simulink model "GHV_open_VarialbeMass_elliposid_toolbox"  (R2023b)
settings: Solver=FixedStepAuto  StartTime=0.0  StopTime=10  FixedStep=0.01  MaxStep=0.001  RelTol=1e-3
InitFcn:
  | run('init.m')
values from neighbouring files (symbols this model uses):
  GHV_cfg = struct()    [GHV_Configuration.m]
undefined symbols (not defined in the file or in its folder): Earth, WGS84
libraries: simulink_extras x3, aerolibasang x3, aerolibtransform2 x2, aerolib6dof2 x1, aerolibatmos2 x1, matrix_library x1, aerolibgravity2 x1
settings Model: SimulationMode=accelerator  Creator=Admin  LastModifiedBy=Admin
settings SolverCC: AllowMultiTaskInputOutput=on  ZeroCrossControl=EnableAll  ZeroCrossAlgorithm=Adaptive  AutoInsertRateTranBlk=on
settings DebuggingCC: IgnoredZcDiagnostic=none

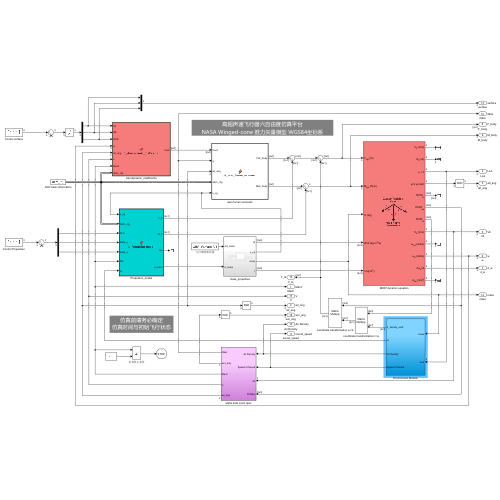
[thumbnail: Simulink's stored preview of the top-level diagram]
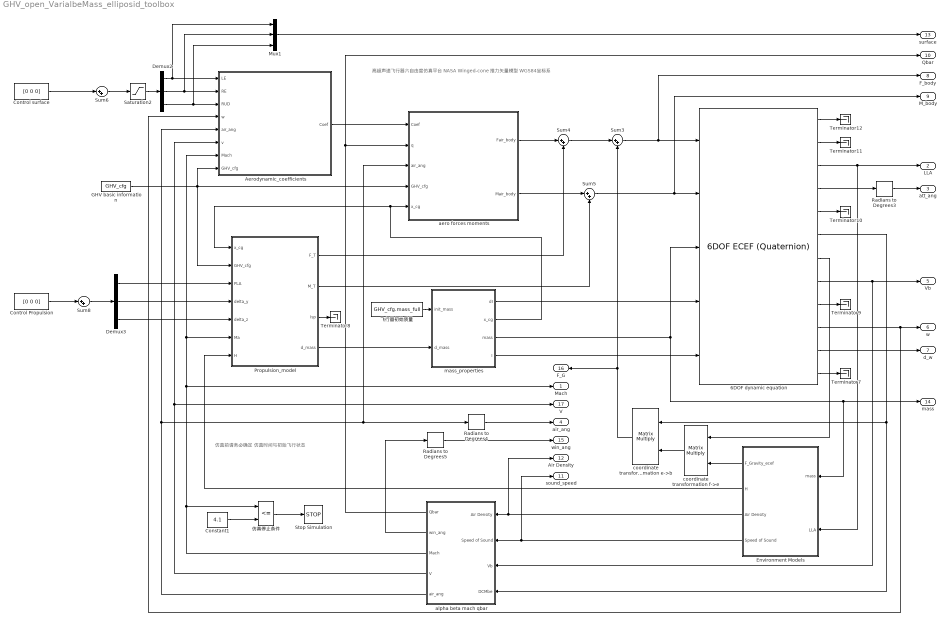
== system GHV_open_VarialbeMass_elliposid_toolbox ==
  note: 高超声速飞行器六自由度仿真平台
      | NASA Winged-cone 推力矢量模型 WGS84坐标系
  note: 仿真前请务必确定
      | 仿真时间与初始飞行状态
  6DOF dynamic equation : aerolib6dof2/6DOF ECEF (Quaternion)  units=Metric (MKS)  mtype=Custom Variable  xg_0=LLA_init  Vm_0=Speed_init  eul_0=Euler_init  pm_0=Omega_init  mass_0=1.0  mass_e=0.5  mass_f=2.0  inertia=eye(3)  inertia_e=eye(3)  inertia_f=2*eye(3)  vre_flag=off  abi_flag=off  ptype=Earth (WGS84)  R=6378137  F=1/298.257223563  w_E=7292115e-11  angle_in=Internal  LPM0=0  quat_statename=''  pm_statename=''  Vm_statename=''  posfixedframe_statename=''  posinertial_statename=''  LPM_statename=''  mass_statename=''
      settings: LibrarySourceBlock=|
      | aerolib6dof2/Custom Variable Mass 6DOF
      | ECEF (Quaternion)
  Aerodynamic_coefficients : MATLAB Function  TreatAsAtomicUnit=on
  Constant1 : Constant  Value=4.1
  Control Propulsion : Constant  Value=[0 0 0]
  Control surface : Constant  Value=[0 0 0]
  Demux2 : Demux  Outputs=3
  Demux3 : Demux  Outputs=3
  Environment Models : Subsystem
  GHV basic information : Constant  Value=GHV_cfg  VectorParams1D=off  OutDataTypeStr=Bus: slBus1
  Mux1 : Mux  Inputs=3
  Propulsion_model : MATLAB Function  TreatAsAtomicUnit=on
  Radians to Degrees3 : simulink_extras/Transformations/Radians to Degrees
  Radians to Degrees4 : simulink_extras/Transformations/Radians to Degrees
  Radians to Degrees5 : simulink_extras/Transformations/Radians to Degrees
  Saturation2 : Saturate  UpperLimit=20  LowerLimit=-20  ZeroCross=off
  Stop Simulation : Stop
  Sum{3..6,8} (5 alike) : Sum  Inputs=|++
  Terminator{7..12} (6 alike) : Terminator
  aero forces moments : MATLAB Function  TreatAsAtomicUnit=on
  alpha beta mach qbar : Subsystem
  coordinate transformation e->b : Product  Multiplication=Matrix(*)
  coordinate transformation f->e : Product  Multiplication=Matrix(*)
  mass_properties : Subsystem
  仿真停止条件 : RelationalOperator  Operator=<=  OutDataTypeStr=boolean  RndMeth=Simplest  InputSameDT=off
  飞行器初始质量 : Constant  Value=GHV_cfg.mass_full
  Mach : Outport  SignalName=Mach
  LLA : Outport  Port=2  SignalName=LLA
  att_ang : Outport  Port=3  SignalName=att_ang
  air_ang : Outport  Port=4  SignalName=air_ang
  Vb : Outport  Port=5  SignalName=Vb
  w : Outport  Port=6  SignalName=w
  d_w : Outport  Port=7  SignalName=d_w
  F_body : Outport  Port=8  SignalName=F_body
  M_body : Outport  Port=9  SignalName=M_body
  Qbar : Outport  Port=10  SignalName=Qbar
  sound_speed : Outport  Port=11  SignalName=sound_speed
  Air Density : Outport  Port=12  SignalName=Air Density
  surface : Outport  Port=13  SignalName=surface
  mass : Outport  Port=14  SignalName=mass
  win_ang : Outport  Port=15  SignalName=win_ang
  F_G : Outport  Port=16  SignalName=F_G
  V : Outport  Port=17  SignalName=V
  wires:
  mass_properties/4(I) -> 6DOF dynamic equation/5
  Propulsion_model/3(Isp) -> Terminator8/1
  alpha beta mach qbar/2(win_ang) -> Radians to Degrees5/1
  Propulsion_model/4(d_mass) -> mass_properties/2(d_mass)
  飞行器初始质量/1 -> mass_properties/1(init_mass)
  仿真停止条件/1 -> Stop Simulation/1
  Demux2/3 -> Aerodynamic_coefficients/3(RUD), Mux1/3
  6DOF dynamic equation/5 -> Terminator10/1
  coordinate transformation e->b/1 -> Sum3/2, F_G/1
  GHV basic information/1 -> aero forces moments/4(GHV_cfg), Propulsion_model/2(GHV_cfg), Aerodynamic_coefficients/8(GHV_cfg)
  6DOF dynamic equation/3 -> LLA/1, Environment Models/2(LLA)
  6DOF dynamic equation/2 -> Terminator11/1
  Environment Models/3(Air Density) -> Air Density/1, alpha beta mach qbar/1(Air Density)
  6DOF dynamic equation/4 -> Radians to Degrees3/1
  Sum8/1 -> Demux3/1
  Demux3/1 -> Propulsion_model/3(PLA)
  alpha beta mach qbar/3(Mach) -> Aerodynamic_coefficients/7(Mach), Propulsion_model/6(Ma), Mach/1, 仿真停止条件/1
  6DOF dynamic equation/8 -> Vb/1, alpha beta mach qbar/3(Vb)
  6DOF dynamic equation/11 -> d_w/1
  Sum4/1 -> Sum3/1
  6DOF dynamic equation/6 -> alpha beta mach qbar/4(DCMbe), coordinate transformation e->b/1
  Propulsion_model/2(M_T) -> Sum5/2
  Sum5/1 -> 6DOF dynamic equation/2, M_body/1
  6DOF dynamic equation/10 -> w/1, Aerodynamic_coefficients/4(w)
  Environment Models/1(F_Gravity_ecef) -> coordinate transformation f->e/2
  mass_properties/1(dI) -> 6DOF dynamic equation/4
  Demux2/1 -> Aerodynamic_coefficients/1(LE), Mux1/1
  Radians to Degrees5/1 -> win_ang/1
  Saturation2/1 -> Demux2/1
  Aerodynamic_coefficients/1(Coef) -> aero forces moments/1(Coef)
  mass_properties/3(mass) -> 6DOF dynamic equation/3, Environment Models/1(mass), mass/1
  Constant1/1 -> 仿真停止条件/2
  Control surface/1 -> Sum6/1
  Sum3/1 -> 6DOF dynamic equation/1, F_body/1
  Radians to Degrees4/1 -> air_ang/1
  alpha beta mach qbar/4(V) -> Aerodynamic_coefficients/6(v), V/1
  alpha beta mach qbar/1(Qbar) -> aero forces moments/2(q), Qbar/1
  Environment Models/2(H) -> Propulsion_model/7(H)
  Demux3/2 -> Propulsion_model/4(delta_y)
  Demux2/2 -> Aerodynamic_coefficients/2(RE), Mux1/2
  6DOF dynamic equation/12 -> Terminator7/1
  Control Propulsion/1 -> Sum8/1
  coordinate transformation f->e/1 -> coordinate transformation e->b/2
  Demux3/3 -> Propulsion_model/5(delta_z)
  Sum6/1 -> Saturation2/1
  Mux1/1 -> surface/1
  Propulsion_model/1(F_T) -> Sum4/2
  aero forces moments/1(Fair_body) -> Sum4/1
  6DOF dynamic equation/9 -> Terminator9/1
  6DOF dynamic equation/7 -> coordinate transformation f->e/1
  aero forces moments/2(Mair_body) -> Sum5/1
  Radians to Degrees3/1 -> att_ang/1
  mass_properties/2(x_cg) -> aero forces moments/5(x_cg), Propulsion_model/1(x_cg)
  Environment Models/4(Speed of Sound) -> sound_speed/1, alpha beta mach qbar/2(Speed of Sound)
  6DOF dynamic equation/1 -> Terminator12/1
  alpha beta mach qbar/5(air_ang) -> Aerodynamic_coefficients/5(air_ang), aero forces moments/3(air_ang), Radians to Degrees4/1

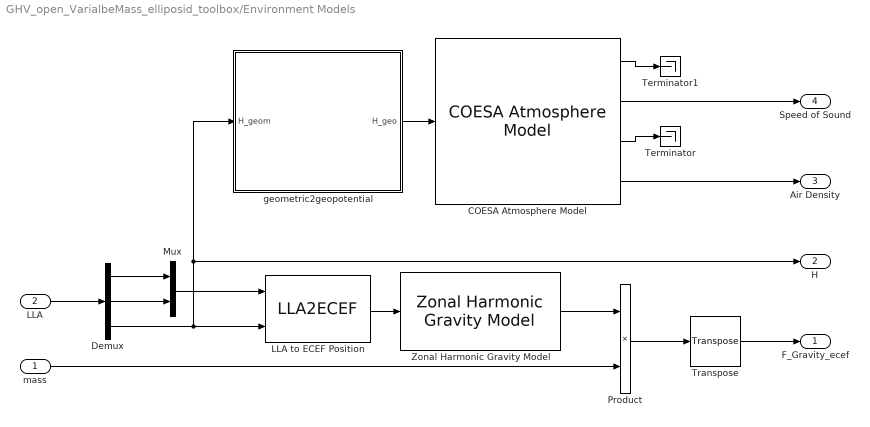
== system GHV_open_VarialbeMass_elliposid_toolbox/Environment Models ==
  mass : Inport
  LLA : Inport  Port=2
  COESA Atmosphere Model : aerolibatmos2/COESA Atmosphere Model  units=Metric (MKS)  spec=1976 COESA-extended U.S. Standard Atmosphere  model=Profile  profile_var=High temperature  profile_percent=1%  profile_alt=5 km (16404 ft)  envelope_var=High temperature  envelope_percent=1%  action=Warning
  Demux : Demux  Outputs=3
  LLA to ECEF Position : LLA2ECEF
  Mux : Mux  Inputs=2
  Product : Product
  Terminator : Terminator
  Terminator1 : Terminator
  Transpose : matrix_library/Transpose
  Zonal Harmonic Gravity Model : aerolibgravity2/Zonal Harmonic Gravity Model  units=Metric (MKS)  degree=2  action=Warning  ptype=Earth  R=6378136.3  GM=398600441500000  jvalue=[1.0826269e-03 -2.5323000e-06 -1.6204000e-06]
  geometric2geopotential : MATLAB Function  TreatAsAtomicUnit=on
  F_Gravity_ecef : Outport
  H : Outport  Port=2
  Air Density : Outport  Port=3
  Speed of Sound : Outport  Port=4
  wires:
  COESA Atmosphere Model/1 -> Terminator1/1
  COESA Atmosphere Model/2 -> Speed of Sound/1
  COESA Atmosphere Model/3 -> Terminator/1
  COESA Atmosphere Model/4 -> Air Density/1
  LLA to ECEF Position/1 -> Zonal Harmonic Gravity Model/1
  Mux/1 -> LLA to ECEF Position/1
  Demux/3 -> geometric2geopotential/1(H_geom), H/1, LLA to ECEF Position/2
  Demux/1 -> Mux/1
  Demux/2 -> Mux/2
  LLA/1 -> Demux/1
  mass/1 -> Product/2
  Zonal Harmonic Gravity Model/1 -> Product/1
  Product/1 -> Transpose/1
  Transpose/1 -> F_Gravity_ecef/1
  geometric2geopotential/1(H_geo) -> COESA Atmosphere Model/1

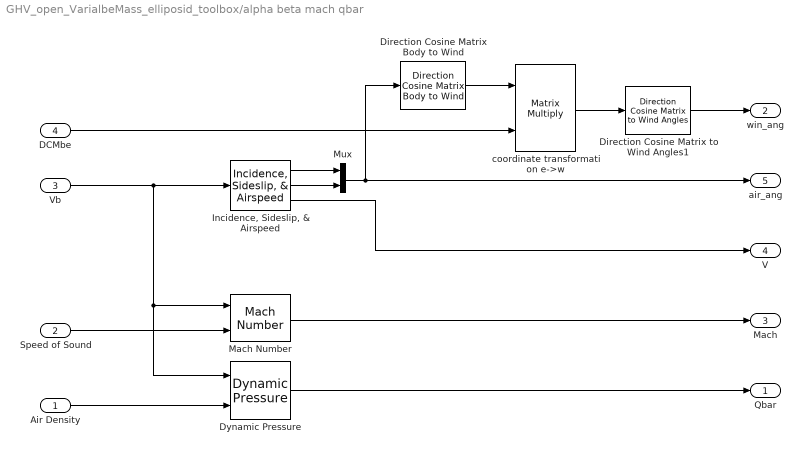
== system GHV_open_VarialbeMass_elliposid_toolbox/alpha beta mach qbar ==
  Air Density : Inport
  Speed of Sound : Inport  Port=2
  Vb : Inport  Port=3
  DCMbe : Inport  Port=4
  Direction Cosine Matrix Body to Wind : aerolibtransform2/Direction Cosine Matrix Body to Wind
  Direction Cosine Matrix to Wind Angles1 : aerolibtransform2/Direction Cosine Matrix to Wind Angles  action=None  tolerance=eps(2)
  Dynamic Pressure : aerolibasang/Dynamic Pressure
  "Incidence, Sideslip, & Airspeed" : aerolibasang/Incidence, Sideslip, & Airspeed
  Mach Number : aerolibasang/Mach Number
  Mux : Mux  Inputs=2
  coordinate transformation e->w : Product  Multiplication=Matrix(*)
  Qbar : Outport
  win_ang : Outport  Port=2
  Mach : Outport  Port=3
  V : Outport  Port=4
  air_ang : Outport  Port=5
  wires:
  Speed of Sound/1 -> Mach Number/2
  Mach Number/1 -> Mach/1
  "Incidence, Sideslip, & Airspeed"/2 -> Mux/2
  Vb/1 -> Dynamic Pressure/1, Mach Number/1, "Incidence, Sideslip, & Airspeed"/1
  Dynamic Pressure/1 -> Qbar/1
  Mux/1 -> Direction Cosine Matrix Body to Wind/1, air_ang/1
  "Incidence, Sideslip, & Airspeed"/1 -> Mux/1
  Air Density/1 -> Dynamic Pressure/2
  "Incidence, Sideslip, & Airspeed"/3 -> V/1
  DCMbe/1 -> coordinate transformation e->w/2
  Direction Cosine Matrix Body to Wind/1 -> coordinate transformation e->w/1
  coordinate transformation e->w/1 -> Direction Cosine Matrix to Wind Angles1/1
  Direction Cosine Matrix to Wind Angles1/1 -> win_ang/1

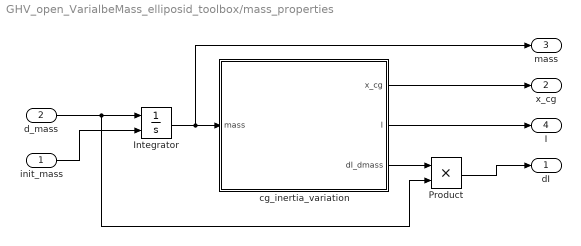
== system GHV_open_VarialbeMass_elliposid_toolbox/mass_properties ==
  init_mass : Inport
  d_mass : Inport  Port=2
  Integrator : Integrator  InitialConditionSource=external
  Product : Product
  cg_inertia_variation : MATLAB Function  TreatAsAtomicUnit=on
  dI : Outport
  x_cg : Outport  Port=2
  mass : Outport  Port=3
  I : Outport  Port=4
  wires:
  Integrator/1 -> mass/1, cg_inertia_variation/1(mass)
  init_mass/1 -> Integrator/2
  cg_inertia_variation/3(dI_dmass) -> Product/1
  d_mass/1 -> Product/2, Integrator/1
  cg_inertia_variation/2(I) -> I/1
  cg_inertia_variation/1(x_cg) -> x_cg/1
  Product/1 -> dI/1

== matlab function GHV_open_VarialbeMass_elliposid_toolbox/Aerodynamic_coefficients ==
  data: LE input; Coef output; RE input; RUD input; w input; air_ang input; v input; Mach input; GHV_cfg input
function Coef = S_Aerodynamic_coefficients(LE, RE, RUD, w, air_ang,v, Mach, GHV_cfg)
    Coef = zeros(6, 1);
    Coef = Aerodynamic_coefficients(LE, RE, RUD, air_ang, v, w, Mach, GHV_cfg);
    Coef = [1;1;1;1;1;1].*Coef;

end

== matlab function GHV_open_VarialbeMass_elliposid_toolbox/Environment Models/geometric2geopotential ==
  data: H_geom input; H_geo output
function H_geo = S_geometric2geopotential(H_geom)

    H_geo = geometric2geopotential(H_geom);

end

== matlab function GHV_open_VarialbeMass_elliposid_toolbox/Propulsion_model ==
  data: F_T output; M_T output; x_cg input; GHV_cfg input; PLA input; delta_y input; delta_z input; Ma input; H input; Isp output; d_mass output
function [F_T,M_T, Isp,  d_mass] = S_Propulsion_model(x_cg, GHV_cfg, PLA, delta_y, delta_z, Ma, H)
    F_T = zeros(3, 1); %#ok<PREALL>
    M_T = zeros(3, 1); %#ok<PREALL>
   [F_T, M_T, Isp, d_mass] = Propulsion_model(PLA, H, Ma, delta_y, delta_z, GHV_cfg, x_cg);

end

== matlab function GHV_open_VarialbeMass_elliposid_toolbox/aero forces moments ==
  data: Coef input; q input; air_ang input; GHV_cfg input; x_cg input; Fair_body output; Mair_body output
function [Fair_body, Mair_body] = S_aero_forces_moments(Coef, q, air_ang, GHV_cfg, x_cg)

    Fair_body = zeros(3, 1); %#ok<PREALL>
    Mair_body = zeros(3, 1); %#ok<PREALL>
    [Fair_body, Mair_body] = aero_forces_moments(Coef, q, GHV_cfg, x_cg, air_ang);

end

== matlab function GHV_open_VarialbeMass_elliposid_toolbox/mass_properties/cg_inertia_variation ==
  data: mass input; x_cg output; I output; dI_dmass output
function [x_cg, I, dI_dmass] = S_cg_inertia_variation(mass)

     [x_cg, I, dI_dmass] = cg_inertia_variation(mass);
     
end
